simulink model "MATLAB_TEST"  (R2019b)
settings: Solver=FixedStepDiscrete  StartTime=0  StopTime=50  FixedStep=0.0025  RelTol=1e-3
undefined symbols (not defined in the file): BCM_COM_PROC_P20, BCM_COM_PROC_P20_SFW_R2018b, BCM_COM_PROC_P2_5, BCM_COM_PROC_P2_5_SFW_R2018b, BCM_COM_PROC_P5, BCM_COM_PROC_P5_SFW_R2018b, BCMA_ACCU_PT_Conf_Flt, BCMA_ACCU_PT_Unconf_Flt, BCMA_Antiskid_Off_Sanction, BCMA_Avionics_Conf_Flt, BCMA_BCM_CCDL_Conf_Flt, BCMA_BCM_CCDL_Unconf_Flt, BCMA_BCM_DBCU_INHIBITION_Conf_Flt, BCMA_BCM_DBCU_INHIBITION_Unconf_Flt, BCMA_BCP_ALT_Disp_Sw_Conf_Flt, BCMA_BCP_ALT_Disp_Sw_Unconf_Flt, BCMA_BCP_ALT_SW_ON_CMD_Conf_Flt, BCMA_BCP_ALT_SW_ON_CMD_Unconf_Flt, BCMA_BCP_PARK_OFF_SW_CMD_Conf_Flt, BCMA_BCP_PARK_OFF_SW_CMD_Unconf_Flt, BCMA_CF_BSELV_JCL, BCMA_CF_BSELV_JOP, BCMA_CF_BSELV_OC, BCMA_CF_BSELV_SC, BCMA_CF_LH_SV_JCL, BCMA_CF_LH_SV_JOP, BCMA_CF_LH_SV_OC, BCMA_CF_LH_SV_SC, BCMA_CF_PARK_BRK, BCMA_CF_RESIDUAL_PRESS, BCMA_CF_RH_SV_JCL, BCMA_CF_RH_SV_JOP, BCMA_CF_RH_SV_OC, BCMA_CF_RH_SV_SC, BCMA_CF_SELV_JCL, BCMA_CF_SELV_JOP, BCMA_CF_SELV_OC, BCMA_CF_SELV_SC, BCMA_CF_SV_DRIFT, BCMA_DBCU_ALT_MODE_Conf_Flt, BCMA_DBCU_ALT_MODE_Unconf_Flt, BCMA_DBCU_BRK_ORDER_FAIL_Conf_Flt, BCMA_DBCU_BRK_ORDER_FAIL_Unconf_Flt, BCMA_DBCU_Conf_Flt, BCMA_DBCU_DISPATCH_SW_ON_Conf_Flt, BCMA_DBCU_DISPATCH_SW_ON_Unconf_Flt, BCMA_DBCU_FAILED_Conf_Flt, BCMA_DBCU_FAILED_Unconf_Flt, BCMA_DFCS1_Capsule_Validity, BCMA_DFCS1_Label202_Corrupted, BCMA_DFCS1_Label202_Not_Refreshed, BCMA_DFCS1_Label204_Corrupted, BCMA_DFCS1_Label204_Not_Refreshed, BCMA_DFCS1_Label205_Corrupted, BCMA_DFCS1_Label205_Not_Refreshed, BCMA_DFCS1_Label206_Corrupted, BCMA_DFCS1_Label206_Not_Refreshed, BCMA_DFCS1_Label207_Corrupted, BCMA_DFCS1_Label207_Not_Refreshed, BCMA_DFCS3_Capsule_Validity ... (+762)
libraries: simulink x73, lib_MBD_Control x5
(part 14 of 16)

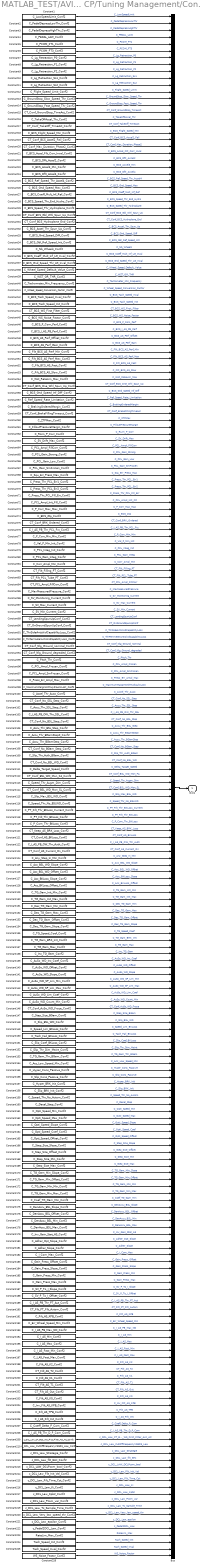
== system MATLAB_TEST/AVIONICS/Brake_Control_Module_Side_A/BCSA Controller CP/Tuning Management/Conf2 ==
  Bus : BusCreator  Inputs=226
  Constant1 : Constant  Value=C_LowSpeedLimit_Conf2
  Constant10 : Constant  Value=C_Lg_Retraction_SL1_Conf2
  Constant100 : Constant  Value=C_Accel_Thr_Auso_Conf2
  Constant101 : Constant  Value=CT_Conf_No_SSL_Step_Conf2
  Constant102 : Constant  Value=C_Accu_Thr_SSL_Step_Conf2
  Constant103 : Constant  Value=C_I_AS_PB_OW_Thr_SSL_Conf2
  Constant104 : Constant  Value=CT_Conf_No_BSL_Step_Conf2
  Constant105 : Constant  Value=C_Accu_Thr_BSL_Step_Conf2
  Constant106 : Constant  Value=C_Accu_Thr_BGamStep0_Conf2
  Constant107 : Constant  Value=C_Accu_Thr_BGamStep_Conf2
  Constant108 : Constant  Value=CT_Conf_No_BGam_Step_Conf2
  Constant109 : Constant  Value=C_Slip_Thr_Auth_BGam_Conf2
  Constant11 : Constant  Value=C_Lg_Retraction_SL2_Conf2
  Constant110 : Constant  Value=CT_Conf_No_BSL_WD_Conf2
  Constant111 : Constant  Value=C_Delta_Target_Speed_Conf2
  Constant112 : Constant  Value=CT_Conf_BSL_WD_Mon_FA_Conf2
  Constant113 : Constant  Value=C_Speed_Thr_Augm_Dim_Conf2
  Constant114 : Constant  Value=CT_Conf_BSL_WD_Mon_SL_Conf2
  Constant115 : Constant  Value=C_Slip_Max_BSL_WD_Conf2
  Constant116 : Constant  Value=C_Speed_Thr_No_BSLWD_Conf2
  Constant117 : Constant  Value=C_PT_Filt_Thr_BKLoss_Current_Conf2
  Constant118 : Constant  Value=C_PT_Filt_Thr_BKLoss_Conf2
  Constant119 : Constant  Value=C_P_Com_Thr_BKLoss_Conf2
  Constant12 : Constant  Value=C_Flight_Speed_Limit_Conf2
  Constant120 : Constant  Value=CT_Keep_AS_BRK_Loss_Conf2
  Constant121 : Constant  Value=CT_Conf_AS_BKLoss_Conf2
  Constant122 : Constant  Value=C_I_AS_PB_OW_Thr_Auth_Conf2
  Constant123 : Constant  Value=CT_Conf_AS_Current_On_Conf2
  Constant124 : Constant  Value=C_Any_Step_In_Min_Conf2
  Constant125 : Constant  Value=C_Acc_BSL_WD_Slope_Conf2
  Constant126 : Constant  Value=C_Acc_BSL_WD_Offset_Conf2
  Constant127 : Constant  Value=C_Acc_BKLoss_Slope_Conf2
  Constant128 : Constant  Value=C_Acc_BKLoss_Offset_Conf2
  Constant129 : Constant  Value=C_TG_Gam_Init_Min_Conf2
  Constant13 : Constant  Value=C_GroundStop_Slow_Speed_Thr_Conf2
  Constant130 : Constant  Value=C_TG_Gam_Init_Max_Conf2
  Constant131 : Constant  Value=C_Dec_TG_Gam_Min_Conf2
  Constant132 : Constant  Value=C_Dec_TG_Gam_Max_Conf2
  Constant133 : Constant  Value=C_Dec_TG_Gam_Offset_Conf2
  Constant134 : Constant  Value=C_Dec_TG_Gam_Slope_Conf2
  Constant135 : Constant  Value=C_TG_Speed_Coef_Conf2
  Constant136 : Constant  Value=C_TG_Gam_BRK_Init_Conf2
  Constant137 : Constant  Value=C_TG_Gam_Max_Conf2
  Constant138 : Constant  Value=C_Inc_TG_Gam_Conf2
  Constant139 : Constant  Value=C_AuSo_WD_Inc_Coef_Conf2
  Constant14 : Constant  Value=C_GroundStop_Fast_Speed_Thr_Conf2
  Constant140 : Constant  Value=C_AuSo_WD_Offset_Conf2
  Constant141 : Constant  Value=C_AuSo_WD_Slope_Conf2
  Constant142 : Constant  Value=C_AuSo_WD_SP_Lim_Min_Conf2
  Constant143 : Constant  Value=C_AuSo_WD_SP_Lim_Max_Conf2
  Constant144 : Constant  Value=C_AuSo_WD_Lim_Coef_Conf2
  Constant145 : Constant  Value=C_AuSo_WD_Count_Min_Conf2
  Constant146 : Constant  Value=CT_Conf_AuSo_WD_Froze_Conf2
  Constant147 : Constant  Value=C_Step_Size_BGam_Conf2
  Constant148 : Constant  Value=C_Slip_BSL_WD_Conf2
  Constant149 : Constant  Value=C_Speed_Lim_BKLoss_Conf2
  Constant15 : Constant  Value=CT_Conf_GroundStop_TimeAct_Conf2
  Constant150 : Constant  Value=C_Tach_Fail_BKLoss_Conf2
  Constant151 : Constant  Value=C_Slip_Coef_BKLoss_Conf2
  Constant152 : Constant  Value=C_Slip_Thr_Dim_Maint_Conf2
  Constant153 : Constant  Value=C_TG_Gam_Thr_BGam_Conf2
  Constant154 : Constant  Value=C_Acc_Low_Speed_Min_Conf2
  Constant155 : Constant  Value=C_Hyper_Cons_Passive_Conf2
  Constant156 : Constant  Value=C_Slip_Cons_Passive_Conf2
  Constant157 : Constant  Value=C_Hyper_BRK_Init_Conf2
  Constant158 : Constant  Value=C_Slip_BRK_Init_Conf2
  Constant159 : Constant  Value=C_Speed_Thr_No_Autom_Conf2
  Constant16 : Constant  Value=C_TakeOffAccel_Thr_Conf2
  Constant160 : Constant  Value=C_Decel_Step_Conf2
  Constant161 : Constant  Value=C_Opti_Speed_Min_Conf2
  Constant162 : Constant  Value=C_Opti_Speed_Max_Conf2
  Constant163 : Constant  Value=C_Opti_Speed_Slope_Conf2
  Constant164 : Constant  Value=C_Opti_Speed_Coef_Conf2
  Constant165 : Constant  Value=C_Opti_Speed_Offset_Conf2
  Constant166 : Constant  Value=C_Step_Size_Slope_Conf2
  Constant167 : Constant  Value=C_Step_Size_Offset_Conf2
  Constant168 : Constant  Value=C_Step_Size_Min_Conf2
  Constant169 : Constant  Value=C_Step_Size_Max_Conf2
  Constant17 : Constant  Value=CT_Conf_TakeOff_TimeAct_Conf2
  Constant170 : Constant  Value=C_TG_Gam_Min_Slope_Conf2
  Constant171 : Constant  Value=C_TG_Gam_Min_Offset_Conf2
  Constant172 : Constant  Value=C_TG_Gam_Min_Min_Conf2
  Constant173 : Constant  Value=C_TG_Gam_Min_Max_Conf2
  Constant174 : Constant  Value=C_Coef_TG_Gam_Min_Conf2
  Constant175 : Constant  Value=C_DenAccu_BSL_Slope_Conf2
  Constant176 : Constant  Value=C_DenAccu_BSL_Offset_Conf2
  Constant177 : Constant  Value=C_DenAccu_BSL_Min_Conf2
  Constant178 : Constant  Value=C_DenAccu_BSL_Max_Conf2
  Constant179 : Constant  Value=C_Inv_Gain_Stat_AS_Conf2
  Constant18 : Constant  Value=C_BCS_Flight_Speed_Min_Conf2
  Constant180 : Constant  Value=C_Adher_Opt_Slope_Conf2
  Constant181 : Constant  Value=C_Adher_Slope_Conf2
  Constant182 : Constant  Value=C_I_Com_Max_Conf2
  Constant183 : Constant  Value=C_Gain_Press_Offset_Conf2
  Constant184 : Constant  Value=C_Gain_Press_Slope_Conf2
  Constant185 : Constant  Value=C_Gain_Press_Min_Conf2
  Constant186 : Constant  Value=C_Gain_Press_Max_Conf2
  Constant187 : Constant  Value=C_SV_P_To_I_Slope_Conf2
  Constant188 : Constant  Value=C_SV_P_To_I_Offset_Conf2
  Constant189 : Constant  Value=C_I_AS_PB_Thr_PT_Aut_Conf2
  Constant19 : Constant  Value=CT_Conf_BCS_Accel2_Fail_Conf2
  Constant190 : Constant  Value=CT_Filt_PT_Filt_Autom_Conf2
  Constant191 : Constant  Value=C_Filt_AS_KPB_Conf2
  Constant192 : Constant  Value=C_Err_Wheel_Speed_Min_Conf2
  Constant193 : Constant  Value=C_I_AS_PB_Max_ND_Conf2
  Constant194 : Constant  Value=C_I_AS_Min_Conf2
  Constant195 : Constant  Value=C_I_AS_Max_Conf2
  Constant196 : Constant  Value=C_I_AS_Fast_Min_Conf2
  Constant197 : Constant  Value=C_I_AS_Fast_Max_Conf2
  Constant198 : Constant  Value=C_Filt_AS_K2_Conf2
  Constant199 : Constant  Value=CT_Filt_AS_T2_Conf2
  Constant2 : Constant  Value=C_PedalDepressLowThr_Conf2
  Constant20 : Constant  Value=CT_Conf_Max_Duration_Phase2_Conf2
  Constant200 : Constant  Value=C_Filt_AS_K1_Conf2
  Constant201 : Constant  Value=CT_Filt_AS_T1_Conf2
  Constant202 : Constant  Value=CT_Filt_AS_Out_Conf2
  Constant203 : Constant  Value=C_Filt_AS_K0_Conf2
  Constant204 : Constant  Value=C_Inv_Filt_AS_KPB_Conf2
  Constant205 : Constant  Value=C_Filt_AS_TPB_Conf2
  Constant206 : Constant  Value=C_I_AS_Filt_Init_Conf2
  Constant207 : Constant  Value=C_Coeff_Delta_P_Com_Conf2
  Constant208 : Constant  Value=C_I_AS_PB_Thr_D_P_Com_Conf2
  Constant209 : Constant  Value=c_DCL_Law_CT_BCS_WS_First_Filter_Acc_AC_Conf2
  Constant21 : Constant  Value=C_BCS_Accel_Filt_Corr_Inval_Conf2
  Constant210 : Constant  Value=c_DCL_Law_CutOffFrequencyVSGRS_Law_Conf2
  Constant211 : Constant  Value=c_DCL_Law_Strategie_Conf2
  Constant212 : Constant  Value=c_DCL_Law_filt_8Hz_Conf2
  Constant213 : Constant  Value=c_DCL_LAW_DCLPcom_bool_Conf2
  Constant214 : Constant  Value=c_DCL_Law_Filt_Init_Val_Conf2
  Constant215 : Constant  Value=c_DCL_Law_Filt_Time_Cst_Conf2
  Constant216 : Constant  Value=c_DCL_Law_Ki_Conf2
  Constant217 : Constant  Value=c_DCL_Law_Kpb2_Conf2
  Constant218 : Constant  Value=c_DCL_Law_Pcom_var_Conf2
  Constant219 : Constant  Value=c_DCL_Law_Ts_Sample_Time_Conf2
  Constant22 : Constant  Value=C_BCS_Dflt_Accel2_Conf2
  Constant220 : Constant  Value=c_DCL_Law_Very_law_speed_thr_Conf2
  Constant221 : Constant  Value=c_DCL_Law_epsilon_Conf2
  Constant222 : Constant  Value=c_Pedal2DCL_Law_Conf2
  Constant223 : Constant  Value=RateLim_Max_Conf2
  Constant224 : Constant  Value=Tach_Speed_Init_Conf2
  Constant225 : Constant  Value=Tach_Speed_Inval_Conf2
  Constant226 : Constant  Value=WS_Noise_Factor_Conf2
  Constant23 : Constant  Value=C_BCS_Accel3_Min_Conf2
  Constant24 : Constant  Value=C_BCS_Dflt_Accel4_Conf2
  Constant25 : Constant  Value=C_BCS_Ref_Speed_Thr_Accel4_Conf2
  Constant26 : Constant  Value=C_BCS_Gnd_Speed_Max_Conf2
  Constant27 : Constant  Value=C_BCS_Coeff_Mult_Inf_Ref_Conf2
  Constant28 : Constant  Value=C_BCS_Speed_Thr_End_Hydro_Conf2
  Constant29 : Constant  Value=C_BCS_Speed_Thr_Hydroplane_Conf2
  Constant3 : Constant  Value=C_PedalDepressHighThr_Conf2
  Constant30 : Constant  Value=CT_Conf_BCS_Gbl_Whl_Spun_Up_Conf2
  Constant31 : Constant  Value=CT_Conf_BCS_Hydroplane_End_Conf2
  Constant32 : Constant  Value=C_BCS_Accel_Thr_Spun_Up_Conf2
  Constant33 : Constant  Value=C_BCS_Gnd_Speed_Diff_Conf2
  Constant34 : Constant  Value=C_BCS_Gbl_Ref_Speed_Init_Conf2
  Constant35 : Constant  Value=C_Nb_Wheels_Conf2
  Constant36 : Constant  Value=C_BCS_Coeff_Mult_Inf_LG_Inval_Conf2
  Constant37 : Constant  Value=C_BCS_Gnd_Speed_Thr_LG_Inval_Conf2
  Constant38 : Constant  Value=C_Wheel_Speed_Default_Value_Conf2
  Constant39 : Constant  Value=C_WST_OR_THR_Conf2
  Constant4 : Constant  Value=C_PEDAL_LAW_Conf2
  Constant40 : Constant  Value=C_Tachometer_Min_Frequency_Conf2
  Constant41 : Constant  Value=C_Wheel_Speed_Conversion_Factor_Conf2
  Constant42 : Constant  Value=C_BCS_Tach_Speed_Inval_Conf2
  Constant43 : Constant  Value=C_BCS_Tach_Speed_Init_Conf2
  Constant44 : Constant  Value=CT_BCS_WS_First_Filter_Conf2
  Constant45 : Constant  Value=C_BCS_WS_Noise_Factor_Conf2
  Constant46 : Constant  Value=C_BCS_P_Com_Perf_Conf2
  Constant47 : Constant  Value=C_BCS_I_AS_PB_Perf_Conf2
  Constant48 : Constant  Value=C_BCS_AS_Perf_Offset_Conf2
  Constant49 : Constant  Value=C_BCS_AS_Perf_Gain_Conf2
  Constant5 : Constant  Value=C_PCOM_FT1_Conf2
  Constant50 : Constant  Value=C_Filt_BCS_AS_Perf_Min_Conf2
  Constant51 : Constant  Value=C_Filt_BCS_AS_Perf_Max_Conf2
  Constant52 : Constant  Value=C_Filt_BCS_AS_Fast_Conf2
  Constant53 : Constant  Value=C_Filt_BCS_AS_Slow_Conf2
  Constant54 : Constant  Value=C_Wst_RateLim_Max_Conf2
  Constant55 : Constant  Value=CT_Conf_BCS_One_Whl_Spun_Up_Conf2
  Constant56 : Constant  Value=C_BCS_Gnd_Speed_Inf_Diff_Conf2
  Constant57 : Constant  Value=C_Ref_Speed_Rate_Limitation_Conf2
  Constant58 : Constant  Value=C_BrakingOrderedMargin_Conf2
  Constant59 : Constant  Value=CT_Conf_BrakeFillingTimeout_Conf2
  Constant6 : Constant  Value=C_PCOM_FT3_Conf2
  Constant60 : Constant  Value=C_ZTPMax_Conf2
  Constant61 : Constant  Value=C_FilloutPressureMargin_Conf2
  Constant62 : Constant  Value=C_RLim_P_Corr_Conf2
  Constant63 : Constant  Value=C_SV_Drift_Max_Conf2
  Constant64 : Constant  Value=C_PCL_Ampl_FillCorr_Conf2
  Constant65 : Constant  Value=C_PCL_Gain_Strong_Conf2
  Constant66 : Constant  Value=C_PCL_Gain_Low_Conf2
  Constant67 : Constant  Value=C_PCL_Gain_SmFrozen_Conf2
  Constant68 : Constant  Value=C_Squ_Err_Press_Max_Conf2
  Constant69 : Constant  Value=C_Press_Thr_PCL_Err1_Conf2
  Constant7 : Constant  Value=C_Lg_Retraction_P0_Conf2
  Constant70 : Constant  Value=C_Press_Thr_PCL_Err2_Conf2
  Constant71 : Constant  Value=C_Press_Thr_PCL_Fill_Err_Conf2
  Constant72 : Constant  Value=C_PCL_Ampl_Init_Fill_Conf2
  Constant73 : Constant  Value=C_P_Corr_Max_Max_Conf2
  Constant74 : Constant  Value=C_BCS_Ztp_Conf2
  Constant75 : Constant  Value=CT_Conf_BRK_Ordered_Conf2
  Constant76 : Constant  Value=C_I_AS_PB_Thr_PCL_Frz_Conf2
  Constant77 : Constant  Value=C_P_Corr_Min_Min_Conf2
  Constant78 : Constant  Value=C_Val_P_Min_Init_Conf2
  Constant79 : Constant  Value=C_PCL_Integ_Init_Conf2
  Constant8 : Constant  Value=C_Lg_Retraction_P1_Conf2
  Constant80 : Constant  Value=C_PCL_Gain_Integ_Conf2
  Constant81 : Constant  Value=C_Corr_Ampl_Min_Conf2
  Constant82 : Constant  Value=CT_Filt_Filling_PT_Conf2
  Constant83 : Constant  Value=CT_Filt_PCL_Tube_PT_Conf2
  Constant84 : Constant  Value=CT_PCL_Ampl_FillCorr_Conf2
  Constant85 : Constant  Value=C_MaxMeasuredPressure_Conf2
  Constant86 : Constant  Value=C_SV_Monitoring_Current_Conf2
  Constant87 : Constant  Value=C_SV_Max_Current_Conf2
  Constant88 : Constant  Value=C_SV_Min_Current_Conf2
  Constant89 : Constant  Value=CT_LandingSpunUpConf_Conf2
  Constant9 : Constant  Value=C_Lg_Retraction_P2_Conf2
  Constant90 : Constant  Value=CT_OnGroundSpunUpConf_Conf2
  Constant91 : Constant  Value=C_ThrSideAntiskidCapabilityLoss_Conf2
  Constant92 : Constant  Value=C_ThrPerimeterAntiskidCapabilityLoss_Conf2
  Constant93 : Constant  Value=CT_Conf_Nlg_Ground_nominal_Conf2
  Constant94 : Constant  Value=CT_Conf_Nlg_Ground_degraded_Conf2
  Constant95 : Constant  Value=C_Pitch_Thr_Conf2
  Constant96 : Constant  Value=C_PCL_Ampl_Frozen_Conf2
  Constant97 : Constant  Value=C_PCL_Ampl_SmFrozen_Conf2
  Constant98 : Constant  Value=C_Press_Err_Ampl_Max_Conf2
  Constant99 : Constant  Value=C_MaximumMarginWithHydraulicLost_Conf2
  Out1 : Outport  VectorParamsAs1DForOutWhenUnconnected=off
  wires:
  Constant1/1 -> Bus/1  "C_LowSpeedLimit"
  Constant2/1 -> Bus/2  "C_PedalDepressLowThr"
  Constant3/1 -> Bus/3  "C_PedalDepressHighThr"
  Constant4/1 -> Bus/4  "C_PEDAL_LAW"
  Constant5/1 -> Bus/5  "C_PCOM_FT1"
  Constant6/1 -> Bus/6  "C_PCOM_FT3"
  Constant7/1 -> Bus/7  "C_Lg_Retraction_P0"
  Constant8/1 -> Bus/8  "C_Lg_Retraction_P1"
  Constant9/1 -> Bus/9  "C_Lg_Retraction_P2"
  Constant10/1 -> Bus/10  "C_Lg_Retraction_SL1"
  Constant11/1 -> Bus/11  "C_Lg_Retraction_SL2"
  Constant12/1 -> Bus/12  "C_Flight_Speed_Limit"
  Constant13/1 -> Bus/13  "C_GroundStop_Slow_Speed_Thr"
  Constant14/1 -> Bus/14  "C_GroundStop_Fast_Speed_Thr"
  Constant15/1 -> Bus/15  "CT_Conf_GroundStop_TimeAct"
  Constant16/1 -> Bus/16  "C_TakeOffAccel_Thr"
  Constant17/1 -> Bus/17  "CT_Conf_TakeOff_TimeAct"
  Constant18/1 -> Bus/18  "C_BCS_Flight_Speed_Min"
  Constant19/1 -> Bus/19  "CT_Conf_BCS_Accel2_Fail"
  Constant20/1 -> Bus/20  "CT_Conf_Max_Duration_Phase2"
  Constant21/1 -> Bus/21  "C_BCS_Accel_Filt_Corr_Inval"
  Constant22/1 -> Bus/22  "C_BCS_Dflt_Accel2"
  Constant23/1 -> Bus/23  "C_BCS_Accel3_Min"
  Constant24/1 -> Bus/24  "C_BCS_Dflt_Accel4"
  Constant25/1 -> Bus/25  "C_BCS_Ref_Speed_Thr_Accel4"
  Constant26/1 -> Bus/26  "C_BCS_Gnd_Speed_Max"
  Constant27/1 -> Bus/27  "C_BCS_Coeff_Mult_Inf_Ref"
  Constant28/1 -> Bus/28  "C_BCS_Speed_Thr_End_Hydro"
  Constant29/1 -> Bus/29  "C_BCS_Speed_Thr_Hydroplane"
  Constant30/1 -> Bus/30  "CT_Conf_BCS_Gbl_Whl_Spun_Up"
  Constant31/1 -> Bus/31  "CT_Conf_BCS_Hydroplane_End"
  Constant32/1 -> Bus/32  "C_BCS_Accel_Thr_Spun_Up"
  Constant33/1 -> Bus/33  "C_BCS_Gnd_Speed_Diff"
  Constant34/1 -> Bus/34  "C_BCS_Gbl_Ref_Speed_Init"
  Constant35/1 -> Bus/35  "C_Nb_Wheels"
  Constant36/1 -> Bus/36  "C_BCS_Coeff_Mult_Inf_LG_Inval"
  Constant37/1 -> Bus/37  "C_BCS_Gnd_Speed_Thr_LG_Inval"
  Constant38/1 -> Bus/38  "C_Wheel_Speed_Default_Value"
  Constant39/1 -> Bus/39  "C_WST_OR_THR"
  Constant40/1 -> Bus/40  "C_Tachometer_Min_Frequency"
  Constant41/1 -> Bus/41  "C_Wheel_Speed_Conversion_Factor"
  Constant42/1 -> Bus/42  "C_BCS_Tach_Speed_Inval"
  Constant43/1 -> Bus/43  "C_BCS_Tach_Speed_Init"
  Constant44/1 -> Bus/44  "CT_BCS_WS_First_Filter"
  Constant45/1 -> Bus/45  "C_BCS_WS_Noise_Factor"
  Constant46/1 -> Bus/46  "C_BCS_P_Com_Perf"
  Constant47/1 -> Bus/47  "C_BCS_I_AS_PB_Perf"
  Constant48/1 -> Bus/48  "C_BCS_AS_Perf_Offset"
  Constant49/1 -> Bus/49  "C_BCS_AS_Perf_Gain"
  Constant50/1 -> Bus/50  "C_Filt_BCS_AS_Perf_Min"
  Constant51/1 -> Bus/51  "C_Filt_BCS_AS_Perf_Max"
  Constant52/1 -> Bus/52  "C_Filt_BCS_AS_Fast"
  Constant53/1 -> Bus/53  "C_Filt_BCS_AS_Slow"
  Constant54/1 -> Bus/54  "C_Wst_RateLim_Max"
  Constant55/1 -> Bus/55  "CT_Conf_BCS_One_Whl_Spun_Up"
  Constant56/1 -> Bus/56  "C_BCS_Gnd_Speed_Inf_Diff"
  Constant57/1 -> Bus/57  "C_Ref_Speed_Rate_Limitation"
  Constant58/1 -> Bus/58  "C_BrakingOrderedMargin"
  Constant59/1 -> Bus/59  "CT_Conf_BrakeFillingTimeout"
  Constant60/1 -> Bus/60  "C_ZTPMax"
  Constant61/1 -> Bus/61  "C_FilloutPressureMargin"
  Constant62/1 -> Bus/62  "C_RLim_P_Corr"
  Constant63/1 -> Bus/63  "C_SV_Drift_Max"
  Constant64/1 -> Bus/64  "C_PCL_Ampl_FillCorr"
  Constant65/1 -> Bus/65  "C_PCL_Gain_Strong"
  Constant66/1 -> Bus/66  "C_PCL_Gain_Low"
  Constant67/1 -> Bus/67  "C_PCL_Gain_SmFrozen"
  Constant68/1 -> Bus/68  "C_Squ_Err_Press_Max"
  Constant69/1 -> Bus/69  "C_Press_Thr_PCL_Err1"
  Constant70/1 -> Bus/70  "C_Press_Thr_PCL_Err2"
  Constant71/1 -> Bus/71  "C_Press_Thr_PCL_Fill_Err"
  Constant72/1 -> Bus/72  "C_PCL_Ampl_Init_Fill"
  Constant73/1 -> Bus/73  "C_P_Corr_Max_Max"
  Constant74/1 -> Bus/74  "C_BCS_Ztp"
  Constant75/1 -> Bus/75  "CT_Conf_BRK_Ordered"
  Constant76/1 -> Bus/76  "C_I_AS_PB_Thr_PCL_Frz"
  Constant77/1 -> Bus/77  "C_P_Corr_Min_Min"
  Constant78/1 -> Bus/78  "C_Val_P_Min_Init"
  Constant79/1 -> Bus/79  "C_PCL_Integ_Init"
  Constant80/1 -> Bus/80  "C_PCL_Gain_Integ"
  Constant81/1 -> Bus/81  "C_Corr_Ampl_Min"
  Constant82/1 -> Bus/82  "CT_Filt_Filling_PT"
  Constant83/1 -> Bus/83  "CT_Filt_PCL_Tube_PT"
  Constant84/1 -> Bus/84  "CT_PCL_Ampl_FillCorr"
  Constant85/1 -> Bus/85  "C_MaxMeasuredPressure"
  Constant86/1 -> Bus/86  "C_SV_Monitoring_Current"
  Constant87/1 -> Bus/87  "C_SV_Max_Current"
  Constant88/1 -> Bus/88  "C_SV_Min_Current"
  Constant89/1 -> Bus/89  "CT_LandingSpunUpConf"
  Constant90/1 -> Bus/90  "CT_OnGroundSpunUpConf"
  Constant91/1 -> Bus/91  "C_ThrSideAntiskidCapabilityLoss"
  Constant92/1 -> Bus/92  "C_ThrPerimeterAntiskidCapabilityLoss"
  Constant93/1 -> Bus/93  "CT_Conf_Nlg_Ground_nominal"
  Constant94/1 -> Bus/94  "CT_Conf_Nlg_Ground_degraded"
  Constant95/1 -> Bus/95  "C_Pitch_Thr"
  Constant96/1 -> Bus/96  "C_PCL_Ampl_Frozen"
  Constant97/1 -> Bus/97  "C_PCL_Ampl_SmFrozen"
  Constant98/1 -> Bus/98  "C_Press_Err_Ampl_Max"
  Constant99/1 -> Bus/99  "C_MaximumMarginWithHydraulicLost"
  Constant100/1 -> Bus/100  "C_Accel_Thr_Auso"
  Constant101/1 -> Bus/101  "CT_Conf_No_SSL_Step"
  Constant102/1 -> Bus/102  "C_Accu_Thr_SSL_Step"
  Constant103/1 -> Bus/103  "C_I_AS_PB_OW_Thr_SSL"
  Constant104/1 -> Bus/104  "CT_Conf_No_BSL_Step"
  Constant105/1 -> Bus/105  "C_Accu_Thr_BSL_Step"
  Constant106/1 -> Bus/106  "C_Accu_Thr_BGamStep0"
  Constant107/1 -> Bus/107  "C_Accu_Thr_BGamStep"
  Constant108/1 -> Bus/108  "CT_Conf_No_BGam_Step"
  Constant109/1 -> Bus/109  "C_Slip_Thr_Auth_BGam"
  Constant110/1 -> Bus/110  "CT_Conf_No_BSL_WD"
  Constant111/1 -> Bus/111  "C_Delta_Target_Speed"
  Constant112/1 -> Bus/112  "CT_Conf_BSL_WD_Mon_FA"
  Constant113/1 -> Bus/113  "C_Speed_Thr_Augm_Dim"
  Constant114/1 -> Bus/114  "CT_Conf_BSL_WD_Mon_SL"
  Constant115/1 -> Bus/115  "C_Slip_Max_BSL_WD"
  Constant116/1 -> Bus/116  "C_Speed_Thr_No_BSLWD"
  Constant117/1 -> Bus/117  "C_PT_Filt_Thr_BKLoss_Current"
  Constant118/1 -> Bus/118  "C_PT_Filt_Thr_BKLoss"
  Constant119/1 -> Bus/119  "C_P_Com_Thr_BKLoss"
  Constant120/1 -> Bus/120  "CT_Keep_AS_BRK_Loss"
  Constant121/1 -> Bus/121  "CT_Conf_AS_BKLoss"
  Constant122/1 -> Bus/122  "C_I_AS_PB_OW_Thr_Auth"
  Constant123/1 -> Bus/123  "CT_Conf_AS_Current_On"
  Constant124/1 -> Bus/124  "C_Any_Step_In_Min"
  Constant125/1 -> Bus/125  "C_Acc_BSL_WD_Slope"
  Constant126/1 -> Bus/126  "C_Acc_BSL_WD_Offset"
  Constant127/1 -> Bus/127  "C_Acc_BKLoss_Slope"
  Constant128/1 -> Bus/128  "C_Acc_BKLoss_Offset"
  Constant129/1 -> Bus/129  "C_TG_Gam_Init_Min"
  Constant130/1 -> Bus/130  "C_TG_Gam_Init_Max"
  Constant131/1 -> Bus/131  "C_Dec_TG_Gam_Min"
  Constant132/1 -> Bus/132  "C_Dec_TG_Gam_Max"
  Constant133/1 -> Bus/133  "C_Dec_TG_Gam_Offset"
  Constant134/1 -> Bus/134  "C_Dec_TG_Gam_Slope"
  Constant135/1 -> Bus/135  "C_TG_Speed_Coef"
  Constant136/1 -> Bus/136  "C_TG_Gam_BRK_Init"
  Constant137/1 -> Bus/137  "C_TG_Gam_Max"
  Constant138/1 -> Bus/138  "C_Inc_TG_Gam"
  Constant139/1 -> Bus/139  "C_AuSo_WD_Inc_Coef"
  Constant140/1 -> Bus/140  "C_AuSo_WD_Offset"
  Constant141/1 -> Bus/141  "C_AuSo_WD_Slope"
  Constant142/1 -> Bus/142  "C_AuSo_WD_SP_Lim_Min"
  Constant143/1 -> Bus/143  "C_AuSo_WD_SP_Lim_Max"
  Constant144/1 -> Bus/144  "C_AuSo_WD_Lim_Coef"
  Constant145/1 -> Bus/145  "C_AuSo_WD_Count_Min"
  Constant146/1 -> Bus/146  "CT_Conf_AuSo_WD_Froze"
  Constant147/1 -> Bus/147  "C_Step_Size_BGam"
  Constant148/1 -> Bus/148  "C_Slip_BSL_WD"
  Constant149/1 -> Bus/149  "C_Speed_Lim_BKLoss"
  Constant150/1 -> Bus/150  "C_Tach_Fail_BKLoss"
  Constant151/1 -> Bus/151  "C_Slip_Coef_BKLoss"
  Constant152/1 -> Bus/152  "C_Slip_Thr_Dim_Maint"
  Constant153/1 -> Bus/153  "C_TG_Gam_Thr_BGam"
  Constant154/1 -> Bus/154  "C_Acc_Low_Speed_Min"
  Constant155/1 -> Bus/155  "C_Hyper_Cons_Passive"
  Constant156/1 -> Bus/156  "C_Slip_Cons_Passive"
  Constant157/1 -> Bus/157  "C_Hyper_BRK_Init"
  Constant158/1 -> Bus/158  "C_Slip_BRK_Init"
  Constant159/1 -> Bus/159  "C_Speed_Thr_No_Autom"
  Constant160/1 -> Bus/160  "C_Decel_Step"
  Constant161/1 -> Bus/161  "C_Opti_Speed_Min"
  Constant162/1 -> Bus/162  "C_Opti_Speed_Max"
  Constant163/1 -> Bus/163  "C_Opti_Speed_Slope"
  Constant164/1 -> Bus/164  "C_Opti_Speed_Coef"
  Constant165/1 -> Bus/165  "C_Opti_Speed_Offset"
  Constant166/1 -> Bus/166  "C_Step_Size_Slope"
  Constant167/1 -> Bus/167  "C_Step_Size_Offset"
  Constant168/1 -> Bus/168  "C_Step_Size_Min"
  Constant169/1 -> Bus/169  "C_Step_Size_Max"
  Constant170/1 -> Bus/170  "C_TG_Gam_Min_Slope"
  Constant171/1 -> Bus/171  "C_TG_Gam_Min_Offset"
  Constant172/1 -> Bus/172  "C_TG_Gam_Min_Min"
  Constant173/1 -> Bus/173  "C_TG_Gam_Min_Max"
  Constant174/1 -> Bus/174  "C_Coef_TG_Gam_Min"
  Constant175/1 -> Bus/175  "C_DenAccu_BSL_Slope"
  Constant176/1 -> Bus/176  "C_DenAccu_BSL_Offset"
  Constant177/1 -> Bus/177  "C_DenAccu_BSL_Min"
  Constant178/1 -> Bus/178  "C_DenAccu_BSL_Max"
  Constant179/1 -> Bus/179  "C_Inv_Gain_Stat_AS"
  Constant180/1 -> Bus/180  "C_Adher_Opt_Slope"
  Constant181/1 -> Bus/181  "C_Adher_Slope"
  Constant182/1 -> Bus/182  "C_I_Com_Max"
  Constant183/1 -> Bus/183  "C_Gain_Press_Offset"
  Constant184/1 -> Bus/184  "C_Gain_Press_Slope"
  Constant185/1 -> Bus/185  "C_Gain_Press_Min"
  Constant186/1 -> Bus/186  "C_Gain_Press_Max"
  Constant187/1 -> Bus/187  "C_SV_P_To_I_Slope"
  Constant188/1 -> Bus/188  "C_SV_P_To_I_Offset"
  Constant189/1 -> Bus/189  "C_I_AS_PB_Thr_PT_Aut"
  Constant190/1 -> Bus/190  "CT_Filt_PT_Filt_Autom"
  Constant191/1 -> Bus/191  "C_Filt_AS_KPB"
  Constant192/1 -> Bus/192  "C_Err_Wheel_Speed_Min"
  Constant193/1 -> Bus/193  "C_I_AS_PB_Max_ND"
  Constant194/1 -> Bus/194  "C_I_AS_Min"
  Constant195/1 -> Bus/195  "C_I_AS_Max"
  Constant196/1 -> Bus/196  "C_I_AS_Fast_Min"
  Constant197/1 -> Bus/197  "C_I_AS_Fast_Max"
  Constant198/1 -> Bus/198  "C_Filt_AS_K2"
  Constant199/1 -> Bus/199  "CT_Filt_AS_T2"
  Constant200/1 -> Bus/200  "C_Filt_AS_K1"
  Constant201/1 -> Bus/201  "CT_Filt_AS_T1"
  Constant202/1 -> Bus/202  "CT_Filt_AS_Out"
  Constant203/1 -> Bus/203  "C_Filt_AS_K0"
  Constant204/1 -> Bus/204  "C_Inv_Filt_AS_KPB"
  Constant205/1 -> Bus/205  "C_Filt_AS_TPB"
  Constant206/1 -> Bus/206  "C_I_AS_Filt_Init"
  Constant207/1 -> Bus/207  "C_Coeff_Delta_P_Com"
  Constant208/1 -> Bus/208  "C_I_AS_PB_Thr_D_P_Com"
  Constant209/1 -> Bus/209  "c_DCL_Law_CT_BCS_WS_First_Filter_Acc_AC"
  Constant210/1 -> Bus/210  "c_DCL_Law_CutOffFrequencyVSGRS_Law"
  Constant211/1 -> Bus/211  "c_DCL_Law_Strategie"
  Constant212/1 -> Bus/212  "c_DCL_Law_filt_8Hz"
  Constant213/1 -> Bus/213  "c_DCL_LAW_DCLPcom_bool"
  Constant214/1 -> Bus/214  "c_DCL_Law_Filt_Init_Val"
  Constant215/1 -> Bus/215  "c_DCL_Law_Filt_Time_Cst"
  Constant216/1 -> Bus/216  "c_DCL_Law_Ki"
  Constant217/1 -> Bus/217  "c_DCL_Law_Kpb2"
  Constant218/1 -> Bus/218  "c_DCL_Law_Pcom_var"
  Constant219/1 -> Bus/219  "c_DCL_Law_Ts_Sample_Time"
  Constant220/1 -> Bus/220  "c_DCL_Law_Very_law_speed_thr"
  Constant221/1 -> Bus/221  "c_DCL_Law_epsilon"
  Constant222/1 -> Bus/222  "c_Pedal2DCL_Law"
  Constant223/1 -> Bus/223  "RateLim_Max"
  Constant224/1 -> Bus/224  "Tach_Speed_Init"
  Constant225/1 -> Bus/225  "Tach_Speed_Inval"
  Constant226/1 -> Bus/226  "WS_Noise_Factor"
  Bus/1 -> Out1/1
